simulink model "Lab14_simulink"  (R2022b)
settings: Solver=VariableStepAuto  StartTime=0.0  StopTime=czas_symulacji  MaxStep=0.1  RelTol=1e-3
values from neighbouring files (symbols this model uses):
  t0 = 100    [lab14.m]
settings Model: Creator=Dawid  LastModifiedBy=Dawid
settings DataIOCC: ReturnWorkspaceOutputs=off

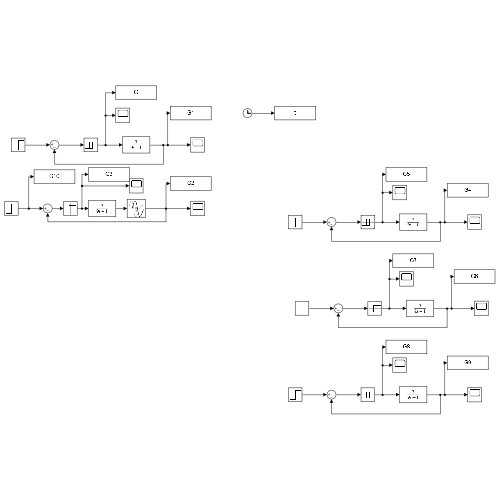
[thumbnail: Simulink's stored preview of the top-level diagram]
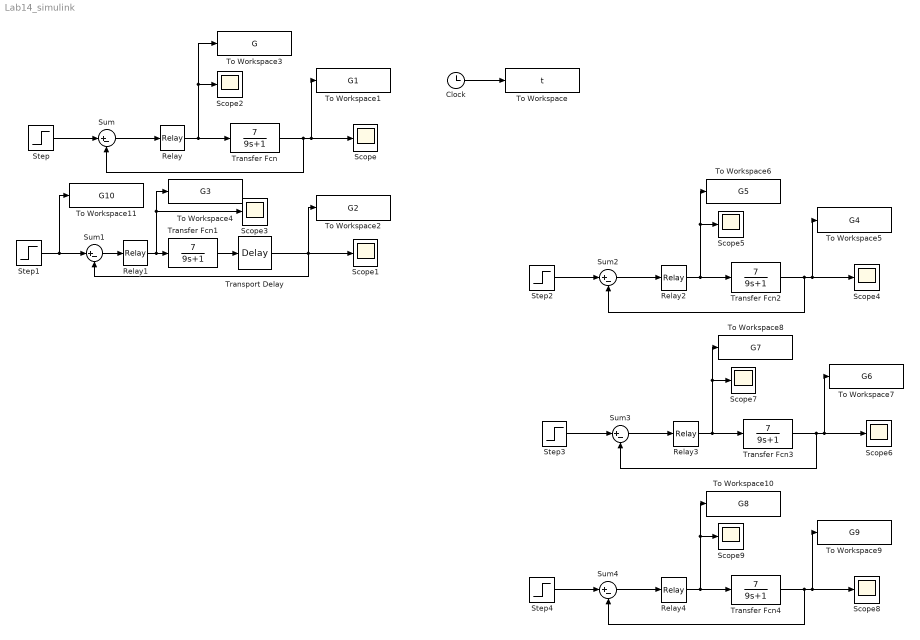
== system Lab14_simulink ==
  Clock : Clock
  Relay : Relay  OnSwitchValue=0.1  OffSwitchValue=-0.1  ZeroCross=off
  Relay1 : Relay  OnSwitchValue=0.1  OffSwitchValue=-0.1  ZeroCross=off
  Relay2 : Relay  OnSwitchValue=0.3  OffSwitchValue=-0.3  ZeroCross=off
  Relay3 : Relay  OnSwitchValue=0.5  OffSwitchValue=-0.5  ZeroCross=off
  Relay4 : Relay  OnSwitchValue=0.7  OffSwitchValue=-0.7  ZeroCross=off
  Scope{,1..9} (10 alike) : Scope
  Step{,1..4} (5 alike) : Step  Time=t0  After=1.5  SampleTime=0
  Sum{,1..4} (5 alike) : Sum  Inputs=|+-
  To Workspace : ToWorkspace  VariableName=t  SaveFormat=Timeseries  SampleTime=-1
  To Workspace1 : ToWorkspace  VariableName=G1  SampleTime=-1
  To Workspace10 : ToWorkspace  VariableName=G8  SampleTime=-1
  To Workspace11 : ToWorkspace  VariableName=G10  SampleTime=-1
  To Workspace2 : ToWorkspace  VariableName=G2  SampleTime=-1
  To Workspace3 : ToWorkspace  VariableName=G  SampleTime=-1
  To Workspace4 : ToWorkspace  VariableName=G3  SampleTime=-1
  To Workspace5 : ToWorkspace  VariableName=G4  SampleTime=-1
  To Workspace6 : ToWorkspace  VariableName=G5  SampleTime=-1
  To Workspace7 : ToWorkspace  VariableName=G6  SampleTime=-1
  To Workspace8 : ToWorkspace  VariableName=G7  SampleTime=-1
  To Workspace9 : ToWorkspace  VariableName=G9  SampleTime=-1
  Transfer Fcn{,1..4} (5 alike) : TransferFcn  Numerator=[7]  Denominator=[9 1]
  Transport Delay : TransportDelay
  wires:
  Step/1 -> Sum/1
  Sum/1 -> Relay/1
  Relay/1 -> To Workspace3/1, Scope2/1, Transfer Fcn/1
  Transfer Fcn/1 -> To Workspace1/1, Scope/1, Sum/2
  Clock/1 -> To Workspace/1
  Step1/1 -> To Workspace11/1, Sum1/1
  Sum1/1 -> Relay1/1
  Relay1/1 -> To Workspace4/1, Scope3/1, Transfer Fcn1/1
  Transfer Fcn1/1 -> Transport Delay/1
  Transport Delay/1 -> Sum1/2, To Workspace2/1, Scope1/1
  Step2/1 -> Sum2/1
  Sum2/1 -> Relay2/1
  Transfer Fcn2/1 -> To Workspace5/1, Scope4/1, Sum2/2
  Relay2/1 -> To Workspace6/1, Scope5/1, Transfer Fcn2/1
  Step3/1 -> Sum3/1
  Sum3/1 -> Relay3/1
  Transfer Fcn3/1 -> To Workspace7/1, Scope6/1, Sum3/2
  Relay3/1 -> To Workspace8/1, Scope7/1, Transfer Fcn3/1
  Step4/1 -> Sum4/1
  Sum4/1 -> Relay4/1
  Transfer Fcn4/1 -> To Workspace9/1, Scope8/1, Sum4/2
  Relay4/1 -> To Workspace10/1, Scope9/1, Transfer Fcn4/1
